simulink library "NormalForce_ul"  (R2020a)
settings: Solver=VariableStepAuto  StartTime=0.0  StopTime=10.0  RelTol=1e-3
libraries: simulink x2
settings Model: Creator=bunce  LastModifiedBy=bunce

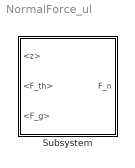
== system NormalForce_ul ==
  Subsystem : Subsystem

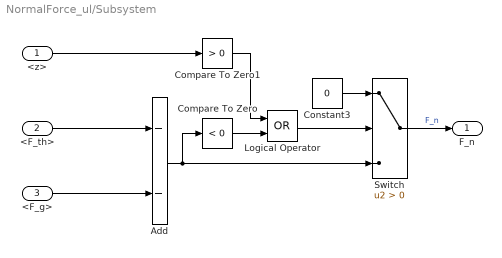
== system NormalForce_ul/Subsystem ==
  <z> : Inport
  <F_th> : Inport  Port=2
  <F_g> : Inport  Port=3
  Add : Sum  Inputs=--
  Compare To Zero : simulink/Logic and Bit Operations/Compare To Zero  relop=<  OutDataTypeStr=boolean
  Compare To Zero1 : simulink/Logic and Bit Operations/Compare To Zero  relop=>  OutDataTypeStr=boolean
  Constant3 : Constant  Value=0
  Logical Operator : Logic  Operator=OR  AllPortsSameDT=off  OutDataTypeStr=boolean
  Switch : Switch  Criteria=u2 > Threshold
  F_n : Outport
  wires:
  <F_g>/1 -> Add/2
  <z>/1 -> Compare To Zero1/1
  Add/1 -> Switch/3, Compare To Zero/1
  Compare To Zero/1 -> Logical Operator/2
  Switch/1 -> F_n/1  "F_n"
  Logical Operator/1 -> Switch/2
  <F_th>/1 -> Add/1
  Compare To Zero1/1 -> Logical Operator/1
  Constant3/1 -> Switch/1
